simulink model "sim_perturbed_od_ekf"  (R2023b)
settings: Solver=VariableStepAuto  StartTime=0.0  StopTime=2*3600  RelTol=1e-3
undefined symbols (not defined in the file or in its folder): earth_grav_param, earth_radius, ekf_sample_time, gps_pos_and_vel_noise_power, gps_pos_noise_power, j2
libraries: simulink x2, sharedTrackingLibrary x2
settings Model: Creator=Atomi  LastModifiedBy=plane

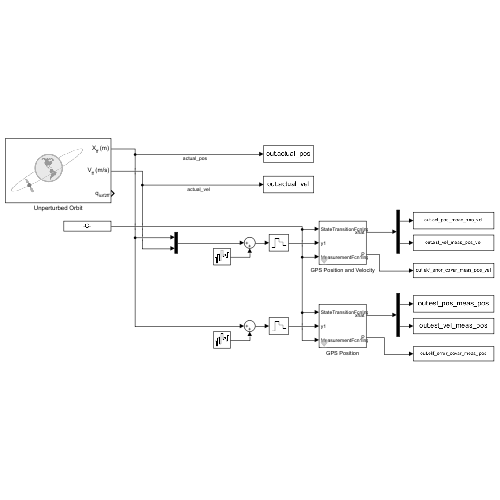
[thumbnail: Simulink's stored preview of the top-level diagram]
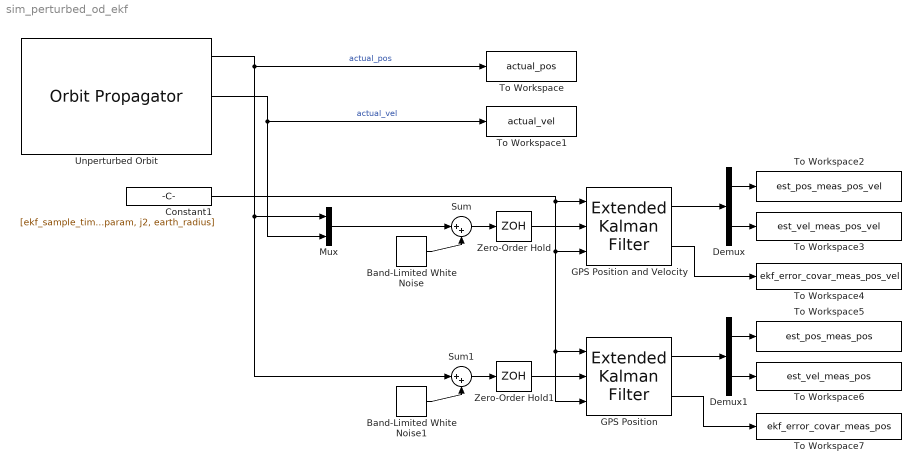
== system sim_perturbed_od_ekf ==
  Band-Limited White Noise : simulink/Sources/Band-Limited White Noise  Cov=gps_pos_and_vel_noise_power/2  Ts=1  seed=[23341]
  Band-Limited White Noise1 : simulink/Sources/Band-Limited White Noise  Cov=gps_pos_noise_power/2  Ts=1  seed=[23341]
  Constant1 : Constant  Value=[ekf_sample_time, earth_grav_param, j2, earth_radius]
  Demux : Demux  Outputs=2
  Demux1 : Demux  Outputs=2
  GPS Position : sharedTrackingLibrary/Extended Kalman Filter  StateTransitionFcn=orbit_state_upd_grav  HasStateTransitionJacobianFcn=off  HasAdditiveProcessNoise=Additive  ProcessNoise=orbit_process_noise_cov  HasTimeVaryingProcessNoise=off  HasStateTransitionFcnExtraArgument=1  InitialState=[3.75E6 4.5E6 -4E6 -3000 6000 4000]  InitialStateCovariance=eye(6,6)  MeasurementFcn1=meas_gps_pos  HasMeasurementJacobianFcn1=off  HasMeasurementEnablePort1=off  HasAdditiveMeasurementNoise1=Additive  MeasurementNoise1=gps_pos_meas_cov  HasTimeVaryingMeasurementNoise1=off  HasMeasurementFcnExtraArgument1=1  HasMeasurementWrapping1=off  MeasurementFcn2=myMeasurementFcn  HasMeasurementJacobianFcn2=off  HasMeasurementEnablePort2=off  HasAdditiveMeasurementNoise2=Additive  MeasurementNoise2=1  HasTimeVaryingMeasurementNoise2=off  HasMeasurementFcnExtraArgument2=0  HasMeasurementWrapping2=off  MeasurementFcn3=myMeasurementFcn  HasMeasurementJacobianFcn3=off  HasMeasurementEnablePort3=off  HasAdditiveMeasurementNoise3=Additive  MeasurementNoise3=1  HasTimeVaryingMeasurementNoise3=off  HasMeasurementFcnExtraArgument3=0  HasMeasurementWrapping3=off  MeasurementFcn4=myMeasurementFcn  HasMeasurementJacobianFcn4=off  HasMeasurementEnablePort4=off  HasAdditiveMeasurementNoise4=Additive  MeasurementNoise4=1  HasTimeVaryingMeasurementNoise4=off  HasMeasurementFcnExtraArgument4=0  HasMeasurementWrapping4=off  MeasurementFcn5=myMeasurementFcn  HasMeasurementJacobianFcn5=off  HasMeasurementEnablePort5=off  HasAdditiveMeasurementNoise5=Additive  MeasurementNoise5=1  HasTimeVaryingMeasurementNoise5=off  HasMeasurementFcnExtraArgument5=0  HasMeasurementWrapping5=off  EnableMultirate=off  StateTransitionFcnSampleTime=1  MeasurementFcn1SampleTime=1  MeasurementFcn2SampleTime=1  MeasurementFcn3SampleTime=1  MeasurementFcn4SampleTime=1  MeasurementFcn5SampleTime=1  UseCurrentEstimator=on  OutputStateCovariance=on  DataType=double  SampleTime=ekf_sample_time  NumberOfMeasurements=1
  GPS Position and Velocity : sharedTrackingLibrary/Extended Kalman Filter  StateTransitionFcn=orbit_state_upd_grav  HasStateTransitionJacobianFcn=off  HasAdditiveProcessNoise=Additive  ProcessNoise=orbit_process_noise_cov  HasTimeVaryingProcessNoise=off  HasStateTransitionFcnExtraArgument=1  InitialState=[3.75E6 4.5E6 -4E6 -3000 6000 4000]  InitialStateCovariance=eye(6,6)  MeasurementFcn1=meas_gps_pos_vel  HasMeasurementJacobianFcn1=off  HasMeasurementEnablePort1=off  HasAdditiveMeasurementNoise1=Additive  MeasurementNoise1=gps_pos_and_vel_meas_cov  HasTimeVaryingMeasurementNoise1=off  HasMeasurementFcnExtraArgument1=1  HasMeasurementWrapping1=off  MeasurementFcn2=myMeasurementFcn  HasMeasurementJacobianFcn2=off  HasMeasurementEnablePort2=off  HasAdditiveMeasurementNoise2=Additive  MeasurementNoise2=1  HasTimeVaryingMeasurementNoise2=off  HasMeasurementFcnExtraArgument2=0  HasMeasurementWrapping2=off  MeasurementFcn3=myMeasurementFcn  HasMeasurementJacobianFcn3=off  HasMeasurementEnablePort3=off  HasAdditiveMeasurementNoise3=Additive  MeasurementNoise3=1  HasTimeVaryingMeasurementNoise3=off  HasMeasurementFcnExtraArgument3=0  HasMeasurementWrapping3=off  MeasurementFcn4=myMeasurementFcn  HasMeasurementJacobianFcn4=off  HasMeasurementEnablePort4=off  HasAdditiveMeasurementNoise4=Additive  MeasurementNoise4=1  HasTimeVaryingMeasurementNoise4=off  HasMeasurementFcnExtraArgument4=0  HasMeasurementWrapping4=off  MeasurementFcn5=myMeasurementFcn  HasMeasurementJacobianFcn5=off  HasMeasurementEnablePort5=off  HasAdditiveMeasurementNoise5=Additive  MeasurementNoise5=1  HasTimeVaryingMeasurementNoise5=off  HasMeasurementFcnExtraArgument5=0  HasMeasurementWrapping5=off  EnableMultirate=off  StateTransitionFcnSampleTime=1  MeasurementFcn1SampleTime=1  MeasurementFcn2SampleTime=1  MeasurementFcn3SampleTime=1  MeasurementFcn4SampleTime=1  MeasurementFcn5SampleTime=1  UseCurrentEstimator=on  OutputStateCovariance=on  DataType=double  SampleTime=ekf_sample_time  NumberOfMeasurements=1
  Mux : Mux  Inputs=2
  Sum : Sum  Inputs=|++
  Sum1 : Sum  Inputs=|++
  To Workspace : ToWorkspace  VariableName=actual_pos  SaveFormat=Timeseries  SampleTime=-1
  To Workspace1 : ToWorkspace  VariableName=actual_vel  SaveFormat=Timeseries  SampleTime=-1
  To Workspace2 : ToWorkspace  VariableName=est_pos_meas_pos_vel  SaveFormat=Timeseries  SampleTime=-1
  To Workspace3 : ToWorkspace  VariableName=est_vel_meas_pos_vel  SaveFormat=Timeseries  SampleTime=-1
  To Workspace4 : ToWorkspace  VariableName=ekf_error_covar_meas_pos_vel  SaveFormat=Timeseries  SampleTime=-1
  To Workspace5 : ToWorkspace  VariableName=est_pos_meas_pos  SaveFormat=Timeseries  SampleTime=-1
  To Workspace6 : ToWorkspace  VariableName=est_vel_meas_pos  SaveFormat=Timeseries  SampleTime=-1
  To Workspace7 : ToWorkspace  VariableName=ekf_error_covar_meas_pos  SaveFormat=Timeseries  SampleTime=-1
  Unperturbed Orbit : OrbitPropagator  propagator=Numerical (high precision)  outportFrame=Fixed-frame  dateOut=off  action=Error  semiMajorAxis=orbit_param.semi_major  eccentricity=orbit_param.eccen  inclination=orbit_param.inclin_deg  raan=orbit_param.raan_deg  argPeriapsis=orbit_param.arg_periapse_deg  trueAnomaly=orbit_param.true_anom_deg  inertialPosition=[3649700.0 3308200.0 -4676600.0]  inertialVelocity=[-2750.8 6666.4 2573.4]  fixedPosition=[-4142689.0 -2676864.7 -4669861.6]  fixedVelocity=[1452.7 -6720.7 2568.1]  customR=3396200  customMu=4.305e13  customJ2=1.0826269e-03  customOmega=4.06125949e-3  outputTransform=on
  Zero-Order Hold : ZeroOrderHold  SampleTime=ekf_sample_time
  Zero-Order Hold1 : ZeroOrderHold  SampleTime=ekf_sample_time
  wires:
  Unperturbed Orbit/2 -> To Workspace1/1, Mux/2  "actual_vel"
  GPS Position and Velocity/1 -> Demux/1
  Demux/1 -> To Workspace2/1
  Demux/2 -> To Workspace3/1
  GPS Position and Velocity/2 -> To Workspace4/1
  Constant1/1 -> GPS Position/3, GPS Position/1, GPS Position and Velocity/3, GPS Position and Velocity/1
  Zero-Order Hold/1 -> GPS Position and Velocity/2
  Zero-Order Hold1/1 -> GPS Position/2
  Unperturbed Orbit/1 -> To Workspace/1, Sum1/1, Mux/1  "actual_pos"
  Demux1/1 -> To Workspace5/1
  Demux1/2 -> To Workspace6/1
  GPS Position/1 -> Demux1/1
  GPS Position/2 -> To Workspace7/1
  Sum/1 -> Zero-Order Hold/1
  Band-Limited White Noise/1 -> Sum/2
  Mux/1 -> Sum/1
  Sum1/1 -> Zero-Order Hold1/1
  Band-Limited White Noise1/1 -> Sum1/2
